simulink model "Closed_Loop_Two_Swtich_Flyback_v03"  (R2023b)
settings: Solver=VariableStepAuto  StartTime=0.0  StopTime=800e-3  FixedStep=1e-7  MaxStep=1e-6  MinStep=1e-8  RelTol=1e-3
libraries: spsMultimeterLib x9, spsSeriesRLCBranchLib x8, spsDiodeLib x7, spsCurrentMeasurementLib x3, spsMosfetLib x2, spsBistableLib x1, spsBreakerLib x1, spsControlledVoltageSourceLib x1, spsEdgeDetectorLib x1, spsLinearTransformerLib x1, eePowerMeasurement x1, spsVoltageMeasurementLib x1
settings Model: VariantFading=off  Creator=Mohammad  LastModifiedBy=Mohammad Derogarian
settings OptimizationCC: ReuseModelBlockBuffer=off

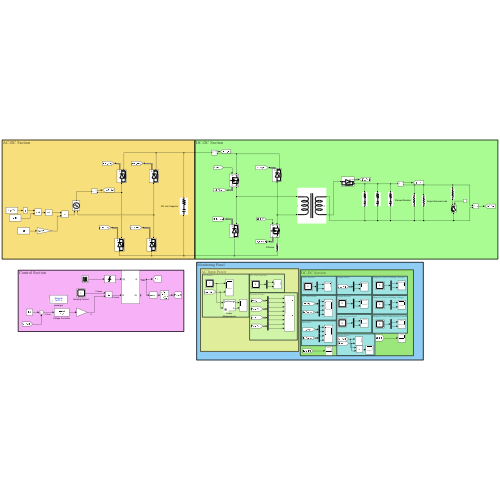
[thumbnail: Simulink's stored preview of the top-level diagram]
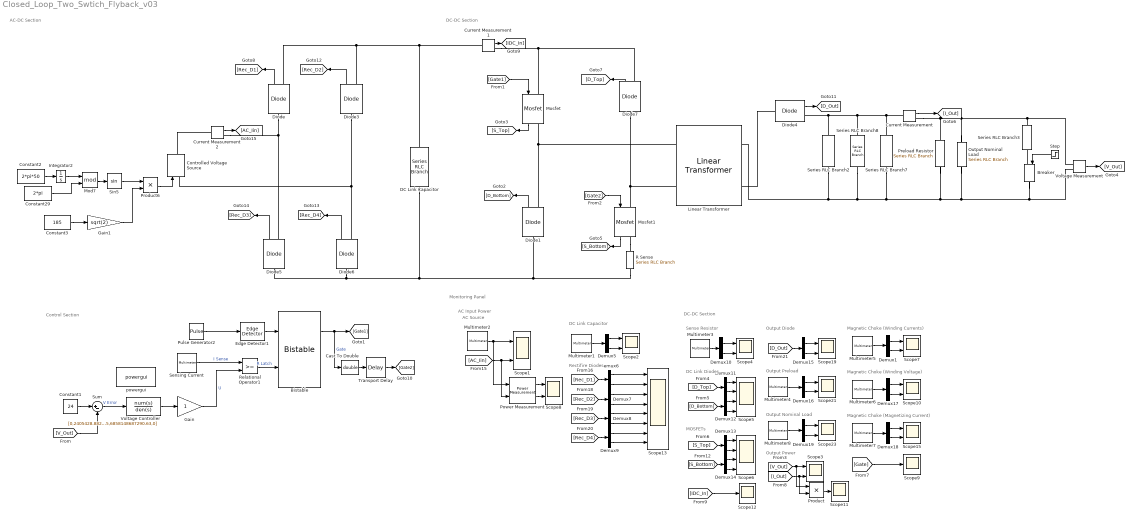
== system Closed_Loop_Two_Swtich_Flyback_v03 ==
  note: AC-DC Section
  note: AC Input Power
  note: AC Source
  note: DC Link Capacitor
  note: Rectifire Diodes
  note: Monitoring Panel
  note: DC-DC Section
  note: DC-DC Section
  note: Sense Resistor
  note: DC Link Diodes
  note: MOSFETs
  note: Output Diode
  note: Output Preload
  note: Magnetic Choke (Winding Currents)
  note: Magnetic Choke (Winding Voltage)
  note: Magnetic Choke (Magnetizing Current)
  note: Output Nominal Load
  note: Control Section
  note: Output Power
  Bistable : spsBistableLib/Bistable  Qpriority=Set  ic=0  Ts=0
      settings: LibrarySourceBlock=sps_lib/Control/Bistable
  Breaker : spsBreakerLib/Breaker  InitialState=0  SwitchingTimes="[1/60  5/60]"  External=on  BreakerResistance=0.01  SnubberResistance=1e6  SnubberCapacitance=inf  Measurements=None  MoreParameters=on  NoBreakLoop=off
  Cast To Double : DataTypeConversion  OutDataTypeStr=double  SaturateOnIntegerOverflow=off  RndMeth=Floor
  Constant1 : Constant  Value=24
  Constant2 : Constant  Value=2*pi*50
  Constant29 : Constant  Value=2*pi
  Constant3 : Constant  Value=185
  Controlled Voltage Source : spsControlledVoltageSourceLib/Controlled Voltage Source  Initialize=on  Source_Type=DC  Amplitude=0  Phase=0  Frequency=0  Measurements=Voltage
  Current Measurement : spsCurrentMeasurementLib/Current Measurement  PhasorSimulation=off  OutputType=Complex  PSBequivalent=0
  Current Measurement1 : spsCurrentMeasurementLib/Current Measurement  PhasorSimulation=off  OutputType=Complex  PSBequivalent=0
  Current Measurement2 : spsCurrentMeasurementLib/Current Measurement  PhasorSimulation=off  OutputType=Complex  PSBequivalent=0
  DC Link Capacitor : spsSeriesRLCBranchLib/Series RLC Branch  LConnTagsString=__new0  RConnTagsString=__new0  BranchType=RC  Resistance=1e-5  Inductance=1e-3  SetiL0=off  InitialCurrent=0  Capacitance=600e-6  Setx0=off  InitialVoltage=0  Measurements=Branch voltage and current
  Demux{1,5..19} (16 alike) : Demux  Outputs=2
  Diode{,1,3,5..7} (6 alike) : spsDiodeLib/Diode  Ron=0.001  Lon=0  Vf=0.8  IC=0  UseSnubber=0  Rs=500  Cs=250e-9  Measurements=on
  Diode4 : spsDiodeLib/Diode  Ron=0.001  Lon=0  Vf=0.1  IC=0  UseSnubber=0  Rs=10e9  Cs=250e-9  Measurements=on
  Edge Detector1 : spsEdgeDetectorLib/Edge Detector  model=Rising  ic=0  Ts=0
      settings: LibrarySourceBlock=sps_lib/Control/Edge Detector
  Gain : Gain
  Gain1 : Gain  Gain=sqrt(2)
  Integrator2 : Integrator
  Linear Transformer : spsLinearTransformerLib/Linear Transformer  UNITS=SI  NominalPower=[500 50e3 ]  winding1=[32 2e-1 10e-6]  winding2=[5 2e-3 1e-6]  ThreeWindings=off  winding3=[1 0 0]  RmLm=[10e6 360e-6]  Measurements=All voltages and currents  DataType=on
  Mod7 : Math  Operator=mod
  Mosfet : spsMosfetLib/Mosfet  Ron=1e-3  Lon=0  Rd=0.01  Vfd=0  IC=0  Rs=1e5  Cs=0.01e-9  Measurements=on
  Mosfet1 : spsMosfetLib/Mosfet  Ron=1e-3  Lon=0  Rd=0.01  Vfd=0  IC=0  Rs=1e5  Cs=0.01e-9  Measurements=on
  Multimeter1 : spsMultimeterLib/Multimeter  L=16  sel=[1 8]  yselected={}  Gain=[1 1]  OutputType=Complex  PlotAtSimulationStop=off  PhasorSimulation=off
  Multimeter2 : spsMultimeterLib/Multimeter  L=16  sel=7  yselected={}  Gain=1  OutputType=Complex  PlotAtSimulationStop=off  PhasorSimulation=off
  Multimeter3 : spsMultimeterLib/Multimeter  L=16  sel=[4 11]  yselected={}  Gain=[1 1]  OutputType=Complex  PlotAtSimulationStop=off  PhasorSimulation=off
  Multimeter4 : spsMultimeterLib/Multimeter  L=16  sel=[3 10]  yselected={}  Gain=[1 1]  OutputType=Complex  PlotAtSimulationStop=off  PhasorSimulation=off
  Multimeter5 : spsMultimeterLib/Multimeter  L=16  sel=[12 13]  yselected={}  Gain=[1 1]  OutputType=Complex  PlotAtSimulationStop=off  PhasorSimulation=off
  Multimeter6 : spsMultimeterLib/Multimeter  L=16  sel=[5 6]  yselected={}  Gain=[1 1]  OutputType=Complex  PlotAtSimulationStop=off  PhasorSimulation=off
  Multimeter7 : spsMultimeterLib/Multimeter  L=16  sel=[15 14]  yselected={}  Gain=[1 1]  OutputType=Complex  PlotAtSimulationStop=off  PhasorSimulation=off
  Multimeter8 : spsMultimeterLib/Multimeter  L=16  sel=[2 9]  yselected={}  Gain=[1 1]  OutputType=Complex  PlotAtSimulationStop=off  PhasorSimulation=off
  Output Nominal Load : spsSeriesRLCBranchLib/Series RLC Branch  LConnTagsString=__new0  RConnTagsString=__new0  BranchType=R  Resistance=24/5.5  Inductance=1e-3  SetiL0=off  InitialCurrent=0  Capacitance=1e-6  Setx0=off  InitialVoltage=0  Measurements=Branch voltage and current
  Power Measurement : eePowerMeasurement/Power Measurement  LabelModeActiveChoice=Continuous  F=50  K=[1]  Ts=0
  Preload Resistor : spsSeriesRLCBranchLib/Series RLC Branch  LConnTagsString=__new0  RConnTagsString=__new0  BranchType=R  Resistance=1.2e3  Inductance=1e-3  SetiL0=off  InitialCurrent=0  Capacitance=1e-6  Setx0=off  InitialVoltage=0  Measurements=Branch voltage and current
  Product : Product
  Product6 : Product
  Pulse Generator2 : DiscretePulseGenerator  PulseType=Time based  Period=1/(50e3)
  R Sense : spsSeriesRLCBranchLib/Series RLC Branch  LConnTagsString=__new0  RConnTagsString=__new0  BranchType=R  Resistance=0.1  Inductance=1e-3  SetiL0=off  InitialCurrent=0  Capacitance=1e-6  Setx0=off  InitialVoltage=0  Measurements=Branch voltage and current
  Relational Operator1 : RelationalOperator  OutDataTypeStr=boolean  RndMeth=Simplest  InputSameDT=off
  Scope{1..4,7..8,10,15,19,21,23} (11 alike) : Scope  NumInputPorts=2
  Scope11 : Scope
  Scope12 : Scope
  Scope13 : Scope  NumInputPorts=8
  Scope5 : Scope  NumInputPorts=4
  Scope6 : Scope  NumInputPorts=4
  Scope9 : Scope
  Sensing Current : spsMultimeterLib/Multimeter  L=16  sel=4  yselected={}  Gain=1  OutputType=Complex  PlotAtSimulationStop=off  PhasorSimulation=off
  Series RLC Branch2 : spsSeriesRLCBranchLib/Series RLC Branch  LConnTagsString=__new0  RConnTagsString=__new0  BranchType=RC  Resistance=1e-3  Inductance=1e-3  SetiL0=off  InitialCurrent=0  Capacitance=200e-6  Setx0=off  InitialVoltage=0  Measurements=None
  Series RLC Branch3 : spsSeriesRLCBranchLib/Series RLC Branch  LConnTagsString=__new0  RConnTagsString=__new0  BranchType=R  Resistance=10  Inductance=1e-3  SetiL0=off  InitialCurrent=0  Capacitance=1e-6  Setx0=off  InitialVoltage=0  Measurements=None
  Series RLC Branch7 : spsSeriesRLCBranchLib/Series RLC Branch  LConnTagsString=__new0  RConnTagsString=__new0  BranchType=RC  Resistance=1e-3  Inductance=1e-3  SetiL0=off  InitialCurrent=0  Capacitance=200e-6  Setx0=off  InitialVoltage=0  Measurements=None
  Series RLC Branch8 : spsSeriesRLCBranchLib/Series RLC Branch  LConnTagsString=__new0  RConnTagsString=__new0  BranchType=RC  Resistance=1e-3  Inductance=1e-3  SetiL0=off  InitialCurrent=0  Capacitance=200e-6  Setx0=off  InitialVoltage=0  Measurements=None
  Sin5 : Trigonometry
  Step : Step  Time=500e-3  After=0  SampleTime=0
  Sum : Sum  Inputs=|+-
  Transport Delay : TransportDelay  DelayTime=0.01/(50e3)
  Voltage Controller : TransferFcn  Numerator=[0,2405428.88270523,196101269282.445,2.55302219455268e+15]  Denominator=[1,5745018.87315035,6858148687290.63,0]
  Voltage Measurement : spsVoltageMeasurementLib/Voltage Measurement  PhasorSimulation=off  OutputType=Complex  PSBequivalent=0
  powergui : sps_lib/powergui  Priority=1  SimulationMode=Discrete  SampleTime=1e-7  frequency=60  Iterations=50  frequencyindice=0  Pbase=100e6  ErrMax=1e-4  UnitsV=kV  UnitsW=MW  buscounter=0  FunctionMessages=off  echomessages=off  EnableUseOfTLC=off  CurrentSourceSwitches=off  DisableSnubberDevices=off  DisableRonSwitches=off  DisableVfSwitches=off  DisplayEquations=off  AutomaticDiscreteSolvers=off  SolverType=Tustin/Backward Euler (TBE)  Interpol=off  ExternalGateDelay=off  methode=off  Ts=100  x0status=blocks  SPID=on  SwTol=0  HookPort=off  NonlinearTolerance=1e-4  nMaxIteration=100  ContinueOnMaxIteration=off  RestoreLinks=warning  ResistiveCurrentMeasurement=off  Frange=[0:2:500]  Ylog=off  Xlog=on  ShowGrid=off  save=off  variable=ZData  structure=0  ZoomFFT=off  StartTime=0.0  cycles=1  DisplayStyle=1  fundamental=60  FreqAxis=off  MaxFrequency=1000  frequencyindicesteady=1  RmsSteady=1  display=off
  wires:
  Constant1/1 -> Sum/1
  [V_Out] -> Sum/2
  Sum/1 -> Voltage Controller/1  "V Error"
  Mosfet1/1 -> [S_Bottom]
  Mosfet/1 -> [S_Top]
  Diode1/1 -> [D_Bottom]
  Diode7/1 -> [D_Top]
  Diode4/1 -> [D_Out]
  Voltage Controller/1 -> Gain/1
  [Gate2] -> Mosfet1/1
  Sensing Current/1 -> Relational Operator1/1  "I Sense"
  Gain/1 -> Relational Operator1/2  "U"
  Relational Operator1/1 -> Bistable/2  "R Latch"
  Bistable/1 -> Cast To Double/1, [Gate1]  "Gate"
  Pulse Generator2/1 -> Edge Detector1/1
  Step/1 -> Breaker/1
  Gain1/1 -> Product6/2
  Constant29/1 -> Mod7/2
  Sin5/1 -> Product6/1
  Constant2/1 -> Integrator2/1
  Integrator2/1 -> Mod7/1
  Product6/1 -> Controlled Voltage Source/1
  Constant3/1 -> Gain1/1
  Mod7/1 -> Sin5/1
  Diode/1 -> [Rec_D1]
  Diode3/1 -> [Rec_D2]
  Diode6/1 -> [Rec_D4]
  Diode5/1 -> [Rec_D3]
  Current Measurement2/1 -> [AC_Iin]
  Multimeter1/1 -> Demux5/1
  Demux5/2 -> Scope2/2
  Demux5/1 -> Scope2/1
  Multimeter2/1 -> Scope1/1, Power Measurement/1
  [AC_Iin] -> Scope1/2, Power Measurement/2
  Power Measurement/2 -> Scope8/2
  Power Measurement/1 -> Scope8/1
  [Rec_D1] -> Demux6/1
  Demux6/1 -> Scope13/1
  Demux6/2 -> Scope13/2
  [Rec_D2] -> Demux7/1
  Demux7/1 -> Scope13/3
  Demux7/2 -> Scope13/4
  Demux8/2 -> Scope13/6
  Demux8/1 -> Scope13/5
  Demux9/2 -> Scope13/8
  Demux9/1 -> Scope13/7
  [Rec_D3] -> Demux8/1
  [Rec_D4] -> Demux9/1
  [Gate1] -> Mosfet/1
  Demux10/1 -> Scope4/1
  Demux10/2 -> Scope4/2
  Multimeter3/1 -> Demux10/1
  [D_Top] -> Demux11/1
  [D_Bottom] -> Demux12/1
  Demux11/1 -> Scope5/1
  Demux11/2 -> Scope5/2
  Demux12/1 -> Scope5/3
  Demux12/2 -> Scope5/4
  Demux14/2 -> Scope6/4
  Demux14/1 -> Scope6/3
  Demux13/2 -> Scope6/2
  Demux13/1 -> Scope6/1
  [S_Bottom] -> Demux14/1
  [S_Top] -> Demux13/1
  [D_Out] -> Demux15/1
  Demux15/1 -> Scope19/1
  Demux15/2 -> Scope19/2
  Demux16/2 -> Scope21/2
  Demux16/1 -> Scope21/1
  Multimeter4/1 -> Demux16/1
  Demux1/2 -> Scope7/2
  Demux1/1 -> Scope7/1
  Multimeter5/1 -> Demux1/1
  Multimeter6/1 -> Demux17/1
  Demux17/1 -> Scope10/1
  Demux17/2 -> Scope10/2
  Demux18/2 -> Scope15/2
  Demux18/1 -> Scope15/1
  Multimeter7/1 -> Demux18/1
  Multimeter8/1 -> Demux19/1
  Demux19/1 -> Scope23/1
  Demux19/2 -> Scope23/2
  Edge Detector1/1 -> Bistable/1
  Voltage Measurement/1 -> [V_Out]
  [V_Out] -> Scope3/1, Product/1
  [Gate] -> Scope9/1
  Current Measurement/1 -> [I_Out]
  [I_Out] -> Product/2, Scope3/2
  Product/1 -> Scope11/1
  Current Measurement1/1 -> [IDC_In]
  [IDC_In] -> Scope12/1
  Cast To Double/1 -> Transport Delay/1
  Transport Delay/1 -> [Gate2]
  connections:
  Diode/RConn1 -- Diode3/RConn1 -- DC Link Capacitor/LConn1 -- Current Measurement1/LConn1
  Diode1/RConn1 -- Linear Transformer/LConn1 -- Mosfet/RConn1
  Mosfet1/LConn1 -- Diode7/LConn1 -- Linear Transformer/LConn2
  Diode6/LConn1 -- DC Link Capacitor/RConn1 -- R Sense/RConn1 -- Diode1/LConn1 -- Diode5/LConn1
  Output Nominal Load/RConn1 -- Series RLC Branch8/RConn1 -- Series RLC Branch2/RConn1 -- Linear Transformer/RConn1 -- Series RLC Branch7/RConn1 -- Preload Resistor/RConn1 -- Breaker/RConn1 -- Voltage Measurement/LConn2
  Output Nominal Load/LConn1 -- Voltage Measurement/LConn1 -- Series RLC Branch3/LConn1 -- Preload Resistor/LConn1 -- Current Measurement/RConn1
  Diode4/LConn1 -- Linear Transformer/RConn2
  Mosfet1/RConn1 -- R Sense/LConn1
  Breaker/LConn1 -- Series RLC Branch3/RConn1
  Diode/LConn1 -- Diode5/RConn1 -- Current Measurement2/RConn1
  Diode3/LConn1 -- Controlled Voltage Source/LConn1 -- Diode6/RConn1
  Current Measurement2/LConn1 -- Controlled Voltage Source/RConn1
  Series RLC Branch2/LConn1 -- Current Measurement/LConn1 -- Series RLC Branch7/LConn1 -- Series RLC Branch8/LConn1 -- Diode4/RConn1
  Diode7/RConn1 -- Mosfet/LConn1 -- Current Measurement1/RConn1
